simulink model "zad1_2"  (R2017b)
settings: Solver=VariableStepAuto  StartTime=0.0  StopTime=0  RelTol=1e-3
undefined symbols (not defined in the file): wariancja
libraries: CPOiS_SourcesSinks x6, CPOiS_DataManipulation_IntroduceNoise x4, CPOiS_LinearTransforms x2, CPOiS_Filters x2, CPOiS_DataManipulation_DataTypeConversion x2, CPOiS_General x1
settings Model: Creator=kstefanc  LastModifiedBy=kstefanc

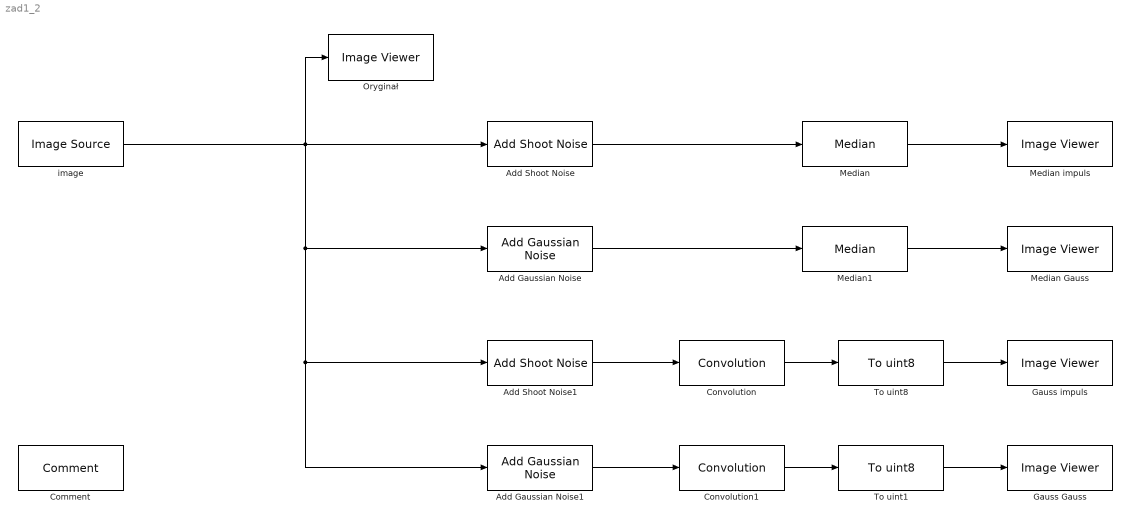
== system zad1_2 ==
  Add Gaussian Noise : CPOiS_DataManipulation_IntroduceNoise/Add Gaussian Noise  Mean=0  Variance=wariancja
      settings: SourceProductName=CPOiS - Digital image and signal processing
  Add Gaussian Noise1 : CPOiS_DataManipulation_IntroduceNoise/Add Gaussian Noise  Mean=0  Variance=wariancja
      settings: SourceProductName=CPOiS - Digital image and signal processing
  Add Shoot Noise : CPOiS_DataManipulation_IntroduceNoise/Add Shoot Noise  Density=impuls
      settings: SourceProductName=CPOiS - Digital image and signal processing
  Add Shoot Noise1 : CPOiS_DataManipulation_IntroduceNoise/Add Shoot Noise  Density=impuls
      settings: SourceProductName=CPOiS - Digital image and signal processing
  Comment : CPOiS_General/Comment
      settings: SourceProductName=CPOiS - Digital image and signal processing
  Convolution : CPOiS_LinearTransforms/Convolution  ConvolutionMatrix=[0,0,0;0,1,0;0,0,0]
      settings: SourceProductName=CPOiS - Digital image and signal processing
  Convolution1 : CPOiS_LinearTransforms/Convolution  ConvolutionMatrix=[0,0,0;0,1,0;0,0,0]
      settings: SourceProductName=CPOiS - Digital image and signal processing
  Gauss Gauss : CPOiS_SourcesSinks/Image Viewer
      settings: SourceProductName=CPOiS - Digital image and signal processing
  Gauss impuls : CPOiS_SourcesSinks/Image Viewer
      settings: SourceProductName=CPOiS - Digital image and signal processing
  Median : CPOiS_Filters/Median  MaskSize=5 x 5
      settings: SourceProductName=CPOiS - Digital image and signal processing
  Median Gauss : CPOiS_SourcesSinks/Image Viewer
      settings: SourceProductName=CPOiS - Digital image and signal processing
  Median impuls : CPOiS_SourcesSinks/Image Viewer
      settings: SourceProductName=CPOiS - Digital image and signal processing
  Median1 : CPOiS_Filters/Median  MaskSize=5 x 5
      settings: SourceProductName=CPOiS - Digital image and signal processing
  Oryginał : CPOiS_SourcesSinks/Image Viewer
      settings: SourceProductName=CPOiS - Digital image and signal processing
  To uint1 : CPOiS_DataManipulation_DataTypeConversion/To uint8
      settings: SourceProductName=CPOiS - Digital image and signal processing
  To uint8 : CPOiS_DataManipulation_DataTypeConversion/To uint8
      settings: SourceProductName=CPOiS - Digital image and signal processing
  image : CPOiS_SourcesSinks/Image Source  FileSelection=gull.png
      settings: SourceProductName=CPOiS - Digital image and signal processing
  wires:
  Add Shoot Noise/1 -> Median/1
  Median/1 -> Median impuls/1
  Median1/1 -> Median Gauss/1
  Add Gaussian Noise/1 -> Median1/1
  Add Shoot Noise1/1 -> Convolution/1
  Add Gaussian Noise1/1 -> Convolution1/1
  image/1 -> Oryginał/1, Add Shoot Noise/1, Add Gaussian Noise/1, Add Shoot Noise1/1, Add Gaussian Noise1/1
  To uint8/1 -> Gauss impuls/1
  Convolution/1 -> To uint8/1
  Convolution1/1 -> To uint1/1
  To uint1/1 -> Gauss Gauss/1
